simulink model "SolutionP145"  (R2018b)
settings: Solver=VariableStepAuto  StartTime=0.0  StopTime=10.0  RelTol=1e-3
values from neighbouring files (symbols this model uses):
  a0 = 1    [SolutionP1.m]    (also in SolutionP22.m; SolutionP31.m)
  a1 = 0.2    [SolutionP1.m]    (also in SolutionP22.m; SolutionP2KalmanFilter.m = -1.5; SolutionP31.m)
  b0 = 1    [SolutionP1.m]    (also in SolutionP22.m; SolutionP2KalmanFilter.m = 0.9; SolutionP31.m)
settings Model: Creator=raphael  LastModifiedBy=raphael

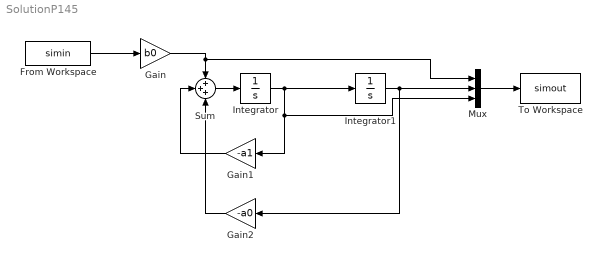
== system SolutionP145 ==
  From Workspace : FromWorkspace  VariableName=simin  SampleTime=0
  Gain : Gain  Gain=b0
  Gain1 : Gain  Gain=-a1
  Gain2 : Gain  Gain=-a0
  Integrator : Integrator
  Integrator1 : Integrator
  Mux : Mux  Inputs=3
  Sum : Sum  Inputs=+++
  To Workspace : ToWorkspace  VariableName=simout  SaveFormat=Timeseries  SampleTime=-1
  wires:
  Sum/1 -> Integrator/1
  Integrator/1 -> Integrator1/1, Mux/3, Gain1/1
  Gain1/1 -> Sum/2
  Gain/1 -> Mux/1, Sum/1
  From Workspace/1 -> Gain/1
  Integrator1/1 -> Gain2/1, Mux/2
  Gain2/1 -> Sum/3
  Mux/1 -> To Workspace/1
